simulink model "Cartesian_regulation_for_the_unicycle"  (R2020a)
settings: Solver=VariableStepAuto  StartTime=0.0  StopTime=10.0  RelTol=1e-3
settings Model: Creator=trinc  LastModifiedBy=ThinkPad

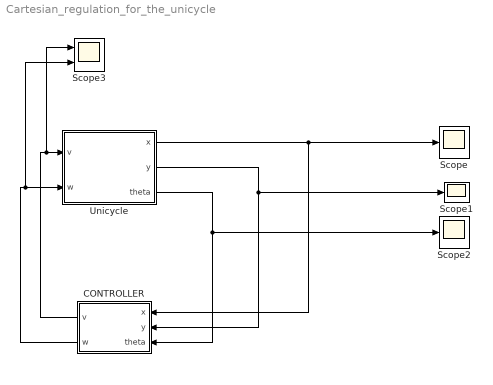
== system Cartesian_regulation_for_the_unicycle ==
  CONTROLLER : MATLAB Function  TreatAsAtomicUnit=on
  Scope : Scope
  Scope1 : Scope
  Scope2 : Scope
  Scope3 : Scope  NumInputPorts=2
  Unicycle : Subsystem
  wires:
  Unicycle/3(theta) -> CONTROLLER/3(theta), Scope2/1
  Unicycle/1(x) -> Scope/1, CONTROLLER/1(x)
  Unicycle/2(y) -> Scope1/1, CONTROLLER/2(y)
  CONTROLLER/2(w) -> Scope3/2, Unicycle/2(w)
  CONTROLLER/1(v) -> Scope3/1, Unicycle/1(v)

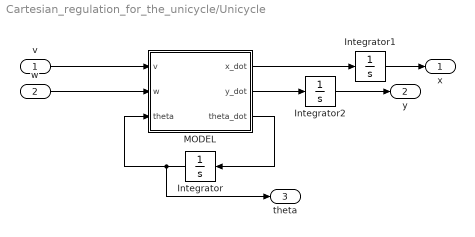
== system Cartesian_regulation_for_the_unicycle/Unicycle ==
  v : Inport
  w : Inport  Port=2
  Integrator : Integrator  InitialCondition=pi/2
  Integrator1 : Integrator  InitialCondition=5
  Integrator2 : Integrator  InitialCondition=2
  MODEL : MATLAB Function  TreatAsAtomicUnit=on
  x : Outport
  y : Outport  Port=2
  theta : Outport  Port=3
  wires:
  Integrator1/1 -> x/1
  Integrator2/1 -> y/1
  Integrator/1 -> theta/1, MODEL/3(theta)
  MODEL/1(x_dot) -> Integrator1/1
  MODEL/2(y_dot) -> Integrator2/1
  w/1 -> MODEL/2(w)
  MODEL/3(theta_dot) -> Integrator/1
  v/1 -> MODEL/1(v)

== matlab function Cartesian_regulation_for_the_unicycle/CONTROLLER ==
  data: x input; v output; w output; y input; theta input
function [v,w] = fcn(x,y,theta)
k_1=1;
k_2=6;
v=-k_1*(x*cos(theta)+y*sin(theta));
w=k_2*(atan2(y,x)+pi-theta);

== matlab function Cartesian_regulation_for_the_unicycle/Unicycle/MODEL ==
  data: v input; x_dot output; w input; y_dot output; theta_dot output; theta input
function [x_dot,y_dot,theta_dot] = fcn(v,w,theta)
x_dot=cos(theta)*v
y_dot=sin(theta)*v
theta_dot=w;
